simulink model "final_integration"  (R2019b)
settings: Solver=FixedStepDiscrete  StartTime=0.0  StopTime=100  FixedStep=0.1  RelTol=1e-3
undefined symbols (not defined in the file): DiscIntNeverNeededParam, gcbh, rmidispblock, sigbuilder_block
libraries: simulink x2
(part 1 of 2)
settings Model: Creator=User  LastModifiedBy=PRACHURJYA
settings OptimizationCC: DefaultParameterBehavior=Inlined  EnhancedBackFolding=on  PassReuseOutputArgsAs=Individual arguments  ZeroExternalMemoryAtStartup=off  ZeroInternalMemoryAtStartup=off  OptimizeBlockOrder=speed  DifferentSizesBufferReuse=on  OptimizationCustomize=off  EfficientTunableParamExpr=on
settings DebuggingCC: ParameterTunabilityLossMsg=error
settings SFSimCC: MATLABDynamicMemAlloc=off
settings RTWCC: SystemTargetFile=ert.tlc  TemplateMakefile=ert_default_tmf  GenerateReport=on  IncludeHyperlinkInReport=on  LaunchReport=on  GenerateTraceInfo=on  GenerateTraceReport=on  GenerateTraceReportSl=on  GenerateTraceReportSf=on  GenerateTraceReportEml=on
settings CodeAppCC: ForceParamTrailComments=on  IgnoreCustomStorageClasses=off  OperatorAnnotations=on  SimulinkDataObjDesc=on  SFDataObjDesc=on  InsertBlockDesc=on
settings ERTTargetCC: TargetLangStandard=C99 (ISO)  GenerateSampleERTMain=on  SupportContinuousTime=on  InlinedParameterPlacement=NonHierarchical  ERTCustomFileTemplate=example_file_process.tlc
settings ConfigComp: CovScope=ReferencedModels  CovMetricSettings=dcmwe  DVTestSuiteOptimization=Auto  DVDetectOutOfBounds=on

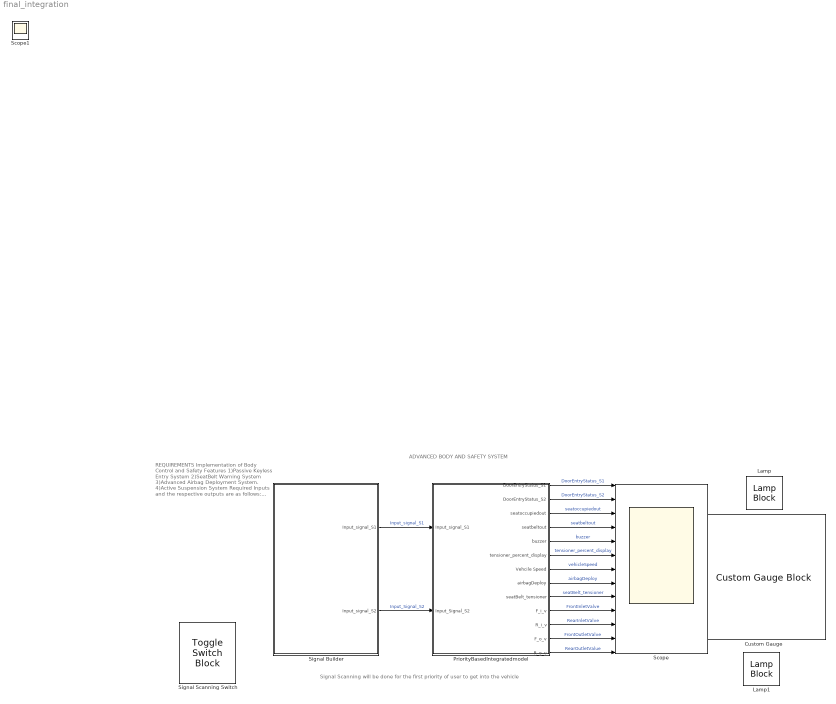
== system final_integration ==
  note: Signal Scanning will be done for the first priority of user to get into the vehicle
  note: REQUIREMENTS
      |
      | Implementation of Body Control and Safety Features
      | 1)Passive Keyless Entry System
      | 2)SeatBelt Warning System
      | 3)Advanced Airbag Deployment System.
      | 4)Active Suspension System
      |
      | Required Inputs and the respective outputs are as follows:
      | 1)Inputs: Input signal_s1
      | Input signal_s2
      | Ignition Status (on/off)
      | Seatbelt status (on/off)
      | Weight Sensor (kg)
      | Distance(cm)
      | Vehicle acceleration(m/s^2).
      | Pressure Input(psi)
      | Mode Status(0/1)
      |
      | 2)Outputs: DoorEntryStatus_S1
      | DoorEntryStatus_S2
      | Seat Occupied Status
      | SeatBelt Status
      | Tensioner Percent
      | Vehicle Speed
      | Airbag Deployment/Steering retraction
      | Seatbelt tensioner status
      | Front/Rear valve signals
  note: ADVANCED BODY AND SAFETY SYSTEM
  Custom Gauge : CustomGaugeBlock  LabelPosition=Bottom  NeedleImage=data:image/svg+xml;base64,PD94bWwgdmVyc2lvbj0iMS4wIiBlbmNvZGluZz0idXRmLTgiPz4KPCEtLSBHZW5lcmF0b3I6IEFkb2JlIElsbHVzdHJhdG9yIDE5LjIuMSwgU1ZHIEV4cG9ydCBQbHVnLUluIC4gU1ZHIFZlcnNpb246IDYuMDAgQnVpbGQgMCkgIC0tPgo8c3ZnIHZlcnNpb249IjEuMSIgeG1sbnM9Imh0dHA6Ly93d3cudzMub3JnLzIwMDAvc3ZnIiB4bWxuczp4bGluaz0iaHR0cDovL3d3dy53My5vcmcvMTk5OS94bGluayIgeD0iMHB4IiB5PSIwcHgiCgkgdmlld0JveD0iMCAwIDIwMCA1MCIgc3R5bGU9ImVuYWJsZS1iYWNrZ3JvdW5kOm5ldyAw ...(+9940 chars)  NeedleXPos=0.3848836610088748  NeedleYPos=0.4819046056238141  NeedleHeight=0.1115133381335879  NeedleWidth=0.18370999021718049  NeedleInitialRotation=-59.94322499147643  BackgroundImage=data:image/svg+xml;base64,PD94bWwgdmVyc2lvbj0iMS4wIiBlbmNvZGluZz0iVVRGLTgiIHN0YW5kYWxvbmU9Im5vIj8+CjwhLS0gR2VuZXJhdG9yOiBBZG9iZSBJbGx1c3RyYXRvciAxOS4yLjEsIFNWRyBFeHBvcnQgUGx1Zy1JbiAuIFNWRyBWZXJzaW9uOiA2LjAwIEJ1aWxkIDApICAtLT4KCjxzdmcKICAgeG1sbnM6ZGM9Imh0dHA6Ly9wdXJsLm9yZy9kYy9lbGVtZW50cy8xLjEvIgogICB4bWxuczpjYz0iaHR0cDovL2NyZWF0aXZlY29tbW9ucy5vcmcvbnMjIgogICB4bWxuczpyZGY9Imh0dHA6Ly93d3cudzMub3JnLzE5OTkvMDIvMjItcmRmLXN5bnRh ...(+9660 chars)  GaugeMax=35  GaugeArcDefined=true  GaugeArcRadius=0.13057749678689773  GaugeArcStrokeWidth=0.03818590063686888  GaugeArcRotation=240.5385250290321  GaugeArcRatio=0.8333333333333  GaugeArcTransparency=0  ValueArcColor=#1759b0  GaugeTickColor=#faf5c8  ScaleColorsJSON=[]  fixedAspectRatio=on  IsLinearGauge=false  GaugeTrackLeft=0.35  GaugeTrackTop=0.35  GaugeTrackHeight=0.1  GaugeTrackWidth=0.3  GaugeTrackRotation=0
  Lamp : LampBlock  LabelPosition=Bottom
  Lamp1 : LampBlock  LabelPosition=Bottom
  PriorityBasedIntegratedmodel : Subsystem
  Scope : Scope  NumInputPorts=13
  Signal Builder : Subsystem  Tag=STV Subsys  LoadFcn=sigbuilder_block('load');  StartFcn=sigbuilder_block('start');  StopFcn=sigbuilder_block('stop');  ClipboardFcn=sigbuilder_block('clipboard');  mask(Sigbuilder block){tuvar=[0:10]}
      mask help: Simulink:masks:SigbuilderBlock_MD
      mask init:
      | if ~strcmp(get_param(bdroot(gcbh),'SimulationStatus'),'stopped') tuvar = sigbuilder_block('maskInit'); end
      settings: CopyFcn=sigbuilder_block('copy');  DeleteFcn=sigbuilder_block('delete');  ModelCloseFcn=sigbuilder_block('modelClose');  PreSaveFcn=sigbuilder_block('preSave');  PauseFcn=sigbuilder_block('pause');  ContinueFcn=sigbuilder_block('continue');  NameChangeFcn=sigbuilder_block('namechange');  OpenFcn=sigbuilder_block('open',[0 30 1152 561.6 ]);  CloseFcn=sigbuilder_block('close');
      mask Display: plot(0, 0, 100, 100,[2, 2, 32, 32, 2], [68, 8, 8, 68, 68],[32, 2], [38, 38], [32, 19, 2],[53, 60, 44], [32, 17, 17, 2],[16, 16, 31, 31]);txt = getActiveGroup(gcbh);text(2, 100, txt,'verticalAlignment', 'top');
  Signal Scanning Switch : ToggleSwitchBlock  LabelPosition=Bottom
      settings: Values={{'Off', 'On'}, [0 1]}
  Scope1 : Scope
  wires:
  Signal Builder/1(Input_signal_S1) -> PriorityBasedIntegratedmodel/1(Input_signal_S1)  "Input_signal_S1"
  Signal Builder/2(Input_signal_S2) -> PriorityBasedIntegratedmodel/2(Input_Signal_S2)  "Input_Signal_S2"
  PriorityBasedIntegratedmodel/1(DoorEntryStatus_S1) -> Scope/1  "DoorEntryStatus_S1"
  PriorityBasedIntegratedmodel/2(DoorEntryStatus_S2) -> Scope/2  "DoorEntryStatus_S2"
  PriorityBasedIntegratedmodel/3(seatoccupiedout) -> Scope/3  "seatoccupiedout"
  PriorityBasedIntegratedmodel/4(seatbeltout) -> Scope/4  "seatbeltout"
  PriorityBasedIntegratedmodel/5(buzzer) -> Scope/5  "buzzer"
  PriorityBasedIntegratedmodel/6(tensioner_percent_display) -> Scope/6  "tensioner_percent_display"
  PriorityBasedIntegratedmodel/7(Vehcile Speed) -> Scope/7  "vehicleSpeed"
  PriorityBasedIntegratedmodel/8(airbagDeploy) -> Scope/8  "airbagDeploy"
  PriorityBasedIntegratedmodel/9(seatBelt_tensioner) -> Scope/9  "seatBelt_tensioner"
  PriorityBasedIntegratedmodel/10(F_i_v) -> Scope/10  "FrontInletValve"
  PriorityBasedIntegratedmodel/11(R_i_v) -> Scope/11  "RearInletValve"
  PriorityBasedIntegratedmodel/12(F_o_v) -> Scope/12  "FrontOutletValve"
  PriorityBasedIntegratedmodel/13(R_o_v) -> Scope/13  "RearOutletValue"

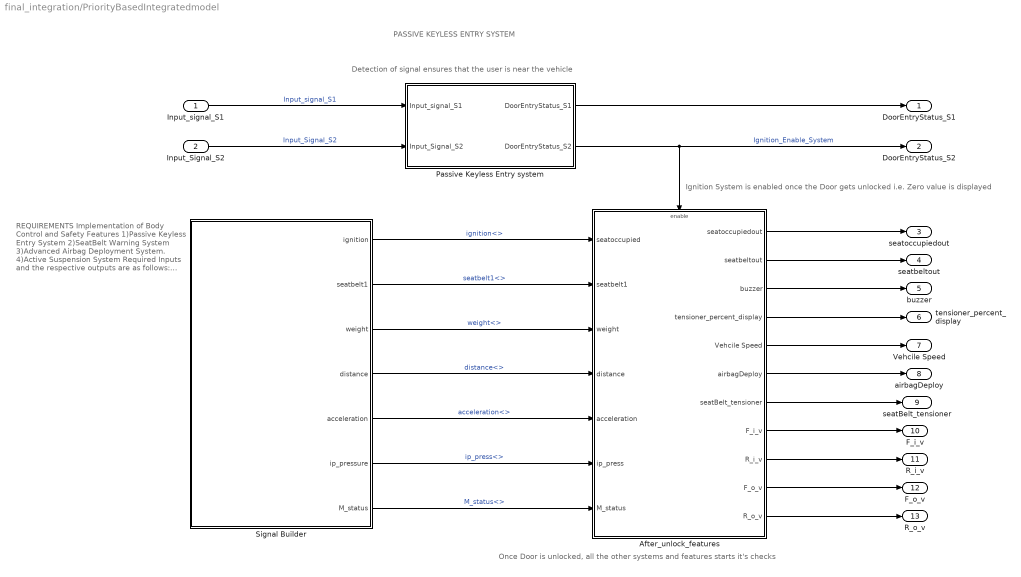
== system final_integration/PriorityBasedIntegratedmodel ==
  note: Once Door is unlocked, all the other systems and features starts it's checks
  note: Ignition System is enabled once the Door gets unlocked i.e. Zero value is displayed
  note: Detection of signal ensures that the user is near the vehicle
  note: PASSIVE KEYLESS ENTRY SYSTEM
  note: REQUIREMENTS
      |
      | Implementation of Body Control and Safety Features
      | 1)Passive Keyless Entry System
      | 2)SeatBelt Warning System
      | 3)Advanced Airbag Deployment System.
      | 4)Active Suspension System
      |
      | Required Inputs and the respective outputs are as follows:
      | 1)Inputs: Input signal_s1
      | Input signal_s2
      | Ignition Status (on/off)
      | Seatbelt status (on/off)
      | Weight Sensor (kg)
      | Distance(cm)
      | Vehicle acceleration(m/s^2).
      | Pressure Input(psi)
      | Mode Status(0/1)
      |
      | 2)Outputs: DoorEntryStatus_S1
      | DoorEntryStatus_S2
      | Seat Occupied Status
      | SeatBelt Status
      | Tensioner Percent
      | Vehicle Speed
      | Airbag Deployment/Steering retraction
      | Seatbelt tensioner status
      | Front/Rear valve signals
  Input_signal_S1 : Inport
  Input_Signal_S2 : Inport  Port=2
  "After_unlock_features " : Subsystem  TreatAsAtomicUnit=on
  Passive Keyless Entry system : Subsystem
  Signal Builder : Subsystem  Tag=STV Subsys  LoadFcn=sigbuilder_block('load');  StartFcn=sigbuilder_block('start');  StopFcn=sigbuilder_block('stop');  ClipboardFcn=sigbuilder_block('clipboard');  mask(Sigbuilder block){tuvar=[0:10]}
      mask help: Simulink:masks:SigbuilderBlock_MD
      mask init:
      | if ~strcmp(get_param(bdroot(gcbh),'SimulationStatus'),'stopped') tuvar = sigbuilder_block('maskInit'); end
      settings: CopyFcn=sigbuilder_block('copy');  DeleteFcn=sigbuilder_block('delete');  ModelCloseFcn=sigbuilder_block('modelClose');  PreSaveFcn=sigbuilder_block('preSave');  PauseFcn=sigbuilder_block('pause');  ContinueFcn=sigbuilder_block('continue');  NameChangeFcn=sigbuilder_block('namechange');  OpenFcn=sigbuilder_block('open',[0 30 1152 561.6 ]);  CloseFcn=sigbuilder_block('close');
      mask Display: plot(0, 0, 100, 100,[2, 2, 32, 32, 2], [68, 8, 8, 68, 68],[32, 2], [38, 38], [32, 19, 2],[53, 60, 44], [32, 17, 17, 2],[16, 16, 31, 31]);txt = getActiveGroup(gcbh);text(2, 100, txt,'verticalAlignment', 'top');
  DoorEntryStatus_S1 : Outport
  DoorEntryStatus_S2 : Outport  Port=2
  seatoccupiedout : Outport  Port=3
  seatbeltout : Outport  Port=4
  buzzer : Outport  Port=5
  tensioner_percent_display : Outport  Port=6
  Vehcile Speed : Outport  Port=7
  airbagDeploy : Outport  Port=8
  seatBelt_tensioner : Outport  Port=9
  F_i_v : Outport  Port=10
  R_i_v : Outport  Port=11
  F_o_v : Outport  Port=12
  R_o_v : Outport  Port=13
  wires:
  "After_unlock_features "/1(seatoccupiedout) -> seatoccupiedout/1
  "After_unlock_features "/2(seatbeltout) -> seatbeltout/1
  "After_unlock_features "/3(buzzer) -> buzzer/1
  "After_unlock_features "/4(tensioner_percent_display) -> tensioner_percent_display/1
  "After_unlock_features "/5(Vehcile Speed) -> Vehcile Speed/1
  "After_unlock_features "/6(airbagDeploy) -> airbagDeploy/1
  "After_unlock_features "/7(seatBelt_tensioner) -> seatBelt_tensioner/1
  "After_unlock_features "/8(F_i_v) -> F_i_v/1
  "After_unlock_features "/9(R_i_v) -> R_i_v/1
  "After_unlock_features "/10(F_o_v) -> F_o_v/1
  "After_unlock_features "/11(R_o_v) -> R_o_v/1
  Passive Keyless Entry system/1(DoorEntryStatus_S1) -> DoorEntryStatus_S1/1
  Input_signal_S1/1 -> Passive Keyless Entry system/1(Input_signal_S1)  "Input_signal_S1"
  Input_Signal_S2/1 -> Passive Keyless Entry system/2(Input_Signal_S2)  "Input_Signal_S2"
  Passive Keyless Entry system/2(DoorEntryStatus_S2) -> "After_unlock_features "/Enable, DoorEntryStatus_S2/1  "Ignition_Enable_System"
  Signal Builder/1(ignition) -> "After_unlock_features "/1(seatoccupied)  "ignition<>"
  Signal Builder/7(M_status) -> "After_unlock_features "/7(M_status)  "M_status<>"
  Signal Builder/2(seatbelt1) -> "After_unlock_features "/2(seatbelt1)  "seatbelt1<>"
  Signal Builder/4(distance) -> "After_unlock_features "/4(distance)  "distance<>"
  Signal Builder/5(acceleration) -> "After_unlock_features "/5(acceleration)  "acceleration<>"
  Signal Builder/6(ip_pressure) -> "After_unlock_features "/6(ip_press)  "ip_press<>"
  Signal Builder/3(weight) -> "After_unlock_features "/3(weight)  "weight<>"

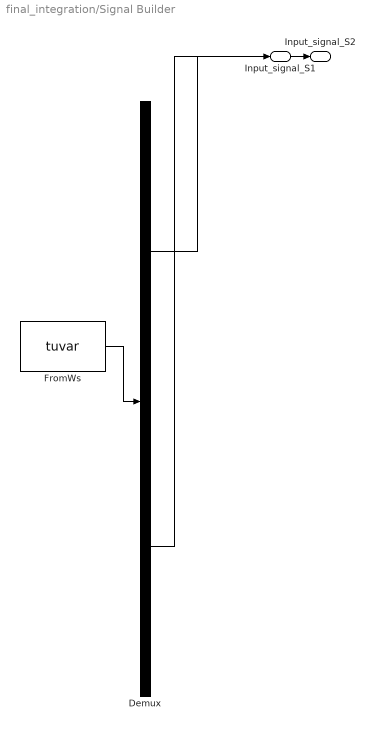
== system final_integration/Signal Builder ==
  Demux : Demux  Tag=STV Demux  Outputs=2
  FromWs : FromWorkspace  Tag=STV FromWs  VariableName=tuvar  SampleTime=0
      SigBuilderData=|
      | common.afterFinalStr = 'Extrapolate'
      | common.sampleTime = 0
      | dataSet.timeRange = [0 100]
      | dataSet.name = 'Passive_entry_system_Signals'
      | sbobj.Groups.Name = 'Passive_entry_system_Signals'
      | sbobj.Groups.Signals(1).Name = 'Input_signal_S1'
      | sbobj.Groups.Signals(1).XData = [0 0.96 7.5 10 100]
      | sbobj.Groups.Signals(1).YData = [0 100 750 1000 1000]
      | sbobj.Groups.Signals(2).Name = 'Input_signal_S2'
      | sbobj.Groups.Signals(2).XData = [0 4 6.16 10 100]
      | sbobj.Groups.Signals(2).YData = [1000 600 384 0 0]
      | sbobj.Groups.TimeRange = [0 100]
  Input_signal_S1 : Outport  Tag=STV Outport
  Input_signal_S2 : Outport  Tag=STV Outport  Port=2
  wires:
  FromWs/1 -> Demux/1
  Demux/1 -> Input_signal_S1/1
  Demux/2 -> Input_signal_S2/1

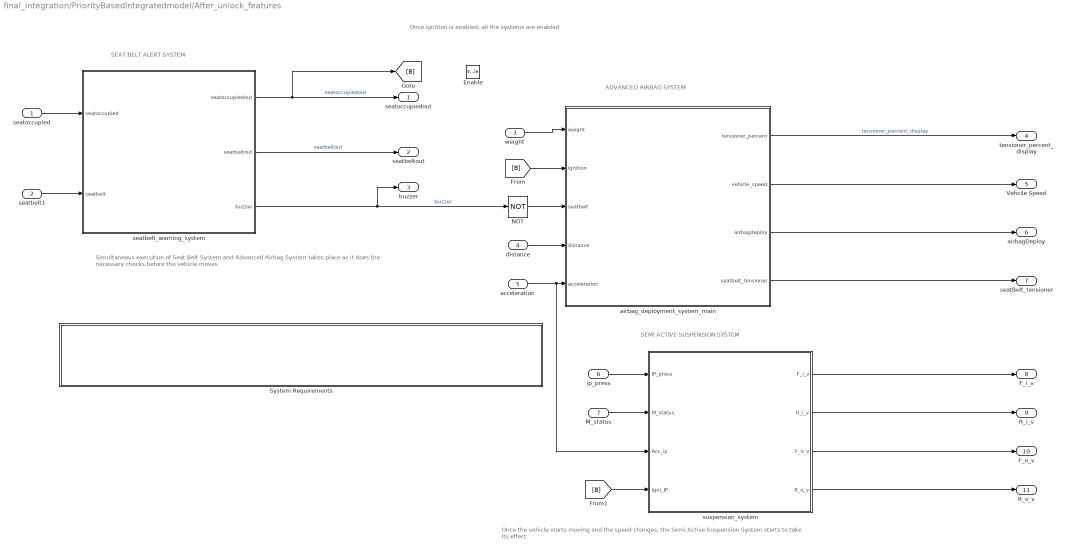
== system final_integration/PriorityBasedIntegratedmodel/After_unlock_features  ==
  note: Once the vehicle starts moving and the speed changes, the Semi Active Suspension System starts to take its effect
  note: Simultaneous execution of Seat Belt System and Advanced Airbag System takes place as
      | it does the necessary checks before the vehicle moves
  note: Once ignition is enabled, all the systems are enabled
  note: SEAT BELT ALERT SYSTEM
  note: ADVANCED AIRBAG SYSTEM
  note: SEMI ACTIVE SUSPENSION SYSTEM
  seatoccupied : Inport
  seatbelt1 : Inport  Port=2
  weight : Inport  Port=3
  distance : Inport  Port=4
  acceleration : Inport  Port=5
  ip_press : Inport  Port=6
  M_status : Inport  Port=7
  Enable : EnablePort
  NOT : Logic  Operator=NOT  IconShape=distinctive  AllPortsSameDT=off  OutDataTypeStr=boolean
  System Requirements : Subsystem  LoadFcn=rmidispblock('load',gcbh)  mask(System Requirements){id=SystemReq, title=System Requirements}
      mask prompts: title "Block Title"
      mask help: Lists the requirements for the current model.
      mask init:
      | id = 'SystemReq';
      | [w,h] = rmidispblock('display',gcbh);
      settings: CopyFcn=rmidispblock('create',gcbh)  DeleteFcn=rmidispblock('delete',gcbh)  ModelCloseFcn=rmidispblock('close',gcbh)  PreSaveFcn=rmidispblock('close',gcbh)  PostSaveFcn=rmidispblock('open',gcbh)  OpenFcn=rmidispblock('open',gcbh)  MoveFcn=rmidispblock('move',gcbh)
      mask Help: helpview(fullfile(docroot,'slrequirements','helptargets.map'),'systemrequirements')
      mask Display: text(746/2,93-4,rmidispblock('title',gcbh),'horizontalAlignment','center','verticalAlignment','top')
  airbag_deployment_system_main : Subsystem
  seatbelt_warning_system : Subsystem
  suspension_system : Subsystem
  seatoccupiedout : Outport
  seatbeltout : Outport  Port=2
  buzzer : Outport  Port=3
  tensioner_percent_display : Outport  Port=4
  Vehcile Speed : Outport  Port=5
  airbagDeploy : Outport  Port=6
  seatBelt_tensioner : Outport  Port=7
  F_i_v : Outport  Port=8
  R_i_v : Outport  Port=9
  F_o_v : Outport  Port=10
  R_o_v : Outport  Port=11
  wires:
  seatbelt1/1 -> seatbelt_warning_system/2(seatbelt)
  seatbelt_warning_system/2(seatbeltout) -> seatbeltout/1  "seatbeltout"
  seatoccupied/1 -> seatbelt_warning_system/1(seatoccupied)
  seatbelt_warning_system/1(seatoccupiedout) -> [B], seatoccupiedout/1  "seatoccupiedout"
  seatbelt_warning_system/3(buzzer) -> buzzer/1, NOT/1  "buzzer"
  distance/1 -> airbag_deployment_system_main/4(distance)
  weight/1 -> airbag_deployment_system_main/1(weight)
  airbag_deployment_system_main/4(seatbelt_tensioner) -> seatBelt_tensioner/1
  NOT/1 -> airbag_deployment_system_main/3(seatbelt)
  airbag_deployment_system_main/3(airbagdeploy) -> airbagDeploy/1
  airbag_deployment_system_main/2(vehicle_speed) -> Vehcile Speed/1
  airbag_deployment_system_main/1(tensioner_percent) -> tensioner_percent_display/1  "tensioner_percent_display"
  [B] -> airbag_deployment_system_main/2(ignition)
  suspension_system/4(R_o_v) -> R_o_v/1
  [B] -> suspension_system/4(Igni_IP)
  suspension_system/2(R_i_v) -> R_i_v/1
  ip_press/1 -> suspension_system/1(IP_press)
  suspension_system/1(F_i_v) -> F_i_v/1
  suspension_system/3(F_o_v) -> F_o_v/1
  M_status/1 -> suspension_system/2(M_status)
  acceleration/1 -> suspension_system/3(Acc_ip), airbag_deployment_system_main/5(acceleration)

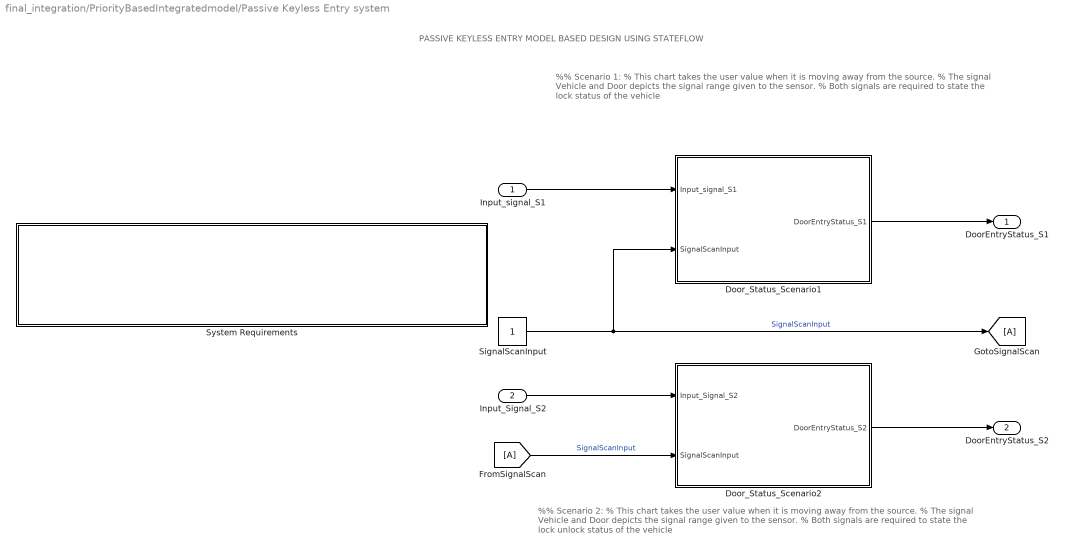
== system final_integration/PriorityBasedIntegratedmodel/Passive Keyless Entry system ==
  note: PASSIVE KEYLESS ENTRY MODEL BASED DESIGN USING STATEFLOW
  note: %% Scenario 1:
      | % This chart takes the user value when it is moving away from the source.
      | % The signal Vehicle and Door depicts the signal range given to the sensor.
      | % Both signals are required to state the lock status of the vehicle
  note: %% Scenario 2:
      | % This chart takes the user value when it is moving away from the source.
      | % The signal Vehicle and Door depicts the signal range given to the sensor.
      | % Both signals are required to state the lock unlock status of the vehicle
  Input_signal_S1 : Inport
  Input_Signal_S2 : Inport  Port=2
  Door_Status_Scenario1 : Stateflow chart  TreatAsAtomicUnit=on
  Door_Status_Scenario2 : Stateflow chart  TreatAsAtomicUnit=on
  SignalScanInput : Constant
  System Requirements : Subsystem  LoadFcn=rmidispblock('load',gcbh)  mask(System Requirements){id=SystemReq, title=System Requirements}
      mask prompts: title "Block Title"
      mask help: Lists the requirements for the current model.
      mask init:
      | id = 'SystemReq';
      | [w,h] = rmidispblock('display',gcbh);
      settings: CopyFcn=rmidispblock('create',gcbh)  DeleteFcn=rmidispblock('delete',gcbh)  ModelCloseFcn=rmidispblock('close',gcbh)  PreSaveFcn=rmidispblock('close',gcbh)  PostSaveFcn=rmidispblock('open',gcbh)  OpenFcn=rmidispblock('open',gcbh)  MoveFcn=rmidispblock('move',gcbh)
      mask Help: helpview(fullfile(docroot,'slrequirements','helptargets.map'),'systemrequirements')
      mask Display: text(511/2,108-4,rmidispblock('title',gcbh),'horizontalAlignment','center','verticalAlignment','top')
  DoorEntryStatus_S1 : Outport
  DoorEntryStatus_S2 : Outport  Port=2
  wires:
  Door_Status_Scenario1/1(DoorEntryStatus_S1) -> DoorEntryStatus_S1/1
  SignalScanInput/1 -> Door_Status_Scenario1/2(SignalScanInput), [A]  "SignalScanInput"
  Door_Status_Scenario2/1(DoorEntryStatus_S2) -> DoorEntryStatus_S2/1
  Input_signal_S1/1 -> Door_Status_Scenario1/1(Input_signal_S1)
  Input_Signal_S2/1 -> Door_Status_Scenario2/1(Input_Signal_S2)
  [A] -> Door_Status_Scenario2/2(SignalScanInput)  "SignalScanInput"

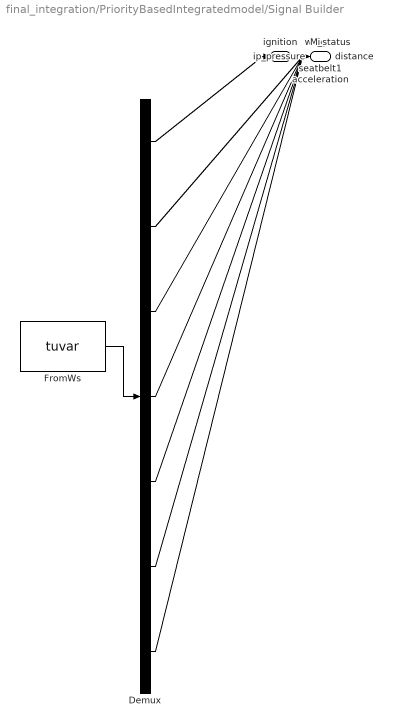
== system final_integration/PriorityBasedIntegratedmodel/Signal Builder ==
  Demux : Demux  Tag=STV Demux  Outputs=7
  FromWs : FromWorkspace  Tag=STV FromWs  VariableName=tuvar  SampleTime=0
      SigBuilderData=|
      | common.afterFinalStr = 'Extrapolate'
      | common.sampleTime = 0
      | dataSet.timeRange = [0 100]
      | dataSet.name = 'Passive_entry_system_Signals'
      | sbobj.Groups.Name = 'Passive_entry_system_Signals'
      | sbobj.Groups.Signals(1).Name = 'ignition'
      | sbobj.Groups.Signals(1).XData = [0 1 2 3 4 5 6 7 7 8 9 9 10 11 11 12 13 13 14 15 16 17 18 19 20 21 22 23 24 25 26 27 28 29 30 31 31.5 31.9 32.3 32.7 33.1 33.5 33.9 34.3 34.7 35.1 35.5 35.9 36.3 36.7 37.1 37.5 37.9 38.3 39 40 41 42 43 44 45 46 47 48 49 50 51 52 53 54 55 56 57 58 59 60 61 62 63 64 65 66 67 68 69 70 71 72 73 74 75 76 77 77 78 79 80 81 82 83 84 85 86 87 88 89 90 91 92 93 94 95 96 97 98 99 100]
      | sbobj.Groups.Signals(1).YData = [0 0 0 1 1 1 1 1 0 0 0 1 1 1 0 0 0 1 1 1 1 1 1 1 1 1 1 1 1 1 1 1 1 1 1 1 0 0 0 0 0 0 0 0 0 0 0 0 0 0 0 0 0 0 0 1 1 1 1 1 1 0 1 1 1 1 0 1 1 0 1 1 1 0 1 1 1 1 1 1 1 1 1 1 0 0 1 0 1 1 1 1 1 0 0 1 1 1 1 1 1 0 1 1 1 1 0 1 1 0 1 1 1 1 1 1 1]
      | sbobj.Groups.Signals(2).Name = 'seatbelt1'
      | sbobj.Groups.Signals(2).XData = [0 1 2 3 3 4 4 5 6 7 7 8 9 10 11 12 13 13 14 15 16 17 18 18 19 20 21 22 23 24 25 26 27 28 29 30 31 31 31.5 31.9 32.3 32.7 33.1 33.5 33.9 34.3 34.7 35.1 35.5 35.9 36.3 36.7 37.1 37.5 37.9 38.3 39 40 40 41 42 43 44 45 46 47 48 49 50 50 51 52 53 54 55 56 57 58 59 60 60 61 62 63 64 65 66 67 68 69 70 71 72 73 73 74 74 75 76 77 77 78 79 79 80 81 82 83 84 85 86 87 88 89 89 90 91 92 93 94 95 95 96 97 98 99 100]
      | sbobj.Groups.Signals(2).YData = [0 0 0 0 1 1 0 0 0 0 1 1 1 1 1 1 1 0 0 0 0 0 0 1 1 1 1 1 1 1 1 1 1 1 1 1 1 0 0 0 1 1 1 1 1 1 1 1 1 1 1 1 1 1 1 1 1 1 0 0 1 1 1 1 1 1 1 1 1 0 0 1 1 1 1 1 1 1 1 1 0 0 1 1 1 1 1 1 1 1 0 1 0 0 1 1 0 0 0 0 1 1 1 0 0 1 1 1 1 1 1 1 1 1 0 0 1 1 1 1 0 1 1 1 1 1 1]
      | sbobj.Groups.Signals(3).Name = 'weight'
      | sbobj.Groups.Signals(3).XData = [0 1 1 2 2 3 3 4 4 5 5 6 6 7 7 8 8 9 9 10 10 11 11 12 12 13 13 14 14 15 15 16 16 17 17 18 18 19 19 20 20 21 21 22 23 24 24 25 25 26 26 27 27 28 28 29 29 30 30 31 31 31.5 31.9 32.3 32.7 33.1 33.5 33.9 34.3 34.7 35.1 35.5 35.9 36.3 36.7 37.1 37.5 37.9 38.3 39 40 41 42 43 44 45 46 47 48 49 50 51 52 52 53 53 54 55 56 57 58 58 59 60 60 61 62 63 63 64 64 65 65 66 66 67 67 68 68 69 70 71 71 72 73 73 74 74 75 75 76 76 77 77 78 78 79 80 81 82 83 84 85 86 87 88 89 90 91 91 92 92 93 94 95 95 96 97 98 99 100]
      | sbobj.Groups.Signals(3).YData = [78 78 68 66 55 55 87 87 43 43 30 30 20 20 10 10 70 70 88 88 99 99 66 66 54 54 34 34 44 44 89 89 86 86 10 10 54 54 44 44 99 99 75 106 106 50 25 25 33 33 26 26 57 57 78 78 57 57 78 78 86 10 10 54 54 44 44 99 99 75 106 106 106 106 50 25 25 33 33 66 55 87 43 30 20 10 70 88 99 66 54 34 44 78 78 86 10 54 44 99 75 106 106 106 50 25 33 66 78 86 10 10 54 54 44 44 99 99 75 106 78 44 99 55 55 87 87 43 43 30 30 20 20 10 10 70 55 87 43 30 20 10 70 88 99 66 54 34 44 78 78 86 10 106 50 86 10 54 44 99 75]
      | sbobj.Groups.Signals(4).Name = 'distance'
      | sbobj.Groups.Signals(4).XData = [0 1 2 3 4 5 6 7 8 9 10 11 12 13 14 15 16 17 18 19 20 21 22 23 24 25 26 27 28 29 30 31 31 31.5 31.9 32.3 32.7 33.1 33.5 33.9 34.3 34.7 35.1 35.5 35.9 36.3 36.7 37.1 37.5 37.9 38.3 39 40 40 41 41 42 42 43 43 44 44 45 45 46 46 47 47 48 48 49 49 50 51 52 53 54 55 56 57 58 59 60 60 61 61 62 62 63 63 64 64 65 65 66 66 67 67 68 68 69 69 70 70 71 71 72 73 74 75 76 77 78 79 79 80 80 81 81 82 82 83 83 84 84 85 85 86 86 87 87 88 88 89 90 91 92 93 94 94 95 95 96 97 98 99 100]
      | sbobj.Groups.Signals(4).YData = [21 22 24 10 18 23 29 50 23 16 13 21 22 19 14 24 15 19 11 22 17 22 24 10 18 23 29 50 23 50 23 23 19 19 11 11 22 22 17 17 22 22 24 24 10 10 18 18 23 23 29 17 17 22 22 24 24 10 10 18 18 23 23 29 29 50 50 23 23 50 50 23 23 19 11 22 17 22 24 10 18 23 29 17 17 22 22 24 24 10 10 18 18 23 23 29 29 50 50 23 23 50 21 22 29 50 24 10 18 23 29 50 23 17 22 22 24 24 10 10 18 18 23 23 29 29 50 50 23 23 50 50 23 23 19 11 22 17 23 29 17 10 18 23 29 50 23]
      | sbobj.Groups.Signals(5).Name = 'acceleration'
      | sbobj.Groups.Signals(5).XData = [0 1 2 3 4 5 6 7 8 9 10 11 12 13 14 15 16 17 18 19 20 21 22 23 24 25 26 27 28 29 30 31 31 31.5 31.9 32.3 32.7 33.1 33.5 33.9 34.3 34.7 35.1 35.5 35.9 36.3 36.7 37.1 37.5 37.9 38.3 39 40 41 42 43 44 45 46 47 48 49 50 51 52 53 54 55 56 57 58 59 60 61 62 63 64 65 66 67 68 69 69 70 70 71 72 73 74 75 76 77 78 79 80 81 82 83 84 85 86 87 88 89 90 91 92 93 94 94 95 95 96 96 97 97 98 98 99 99 100]
      | sbobj.Groups.Signals(5).YData = [9 12 45 54 67 12 47 34 67 23 89 23 52 9 76 13 67 34 90 28 49 12 45 54 67 12 47 34 67 34 67 67 34 34 90 90 90 90 90 90 90 90 90 45 54 54 67 67 12 12 47 12 45 54 67 20 50 34 67 23 89 23 52 76 50 13 67 45 14 88 49 42 45 24 67 12 99 34 67 50 99 9 12 9 12 50 45 54 67 12 47 34 67 45 54 67 20 50 34 67 23 89 23 52 76 50 13 67 42 45 45 99 99 34 34 67 67 50 50 99 99]
      | sbobj.Groups.Signals(6).Name = 'ip_pressure'
      | sbobj.Groups.Signals(6).XData = [0 1 2 3 4 5 6 7 8 9 10 11 12 13 14 15 16 17 18 19 20 21 22 23 24 25 26 27 28 29 30 31 31 31.5 31.9 32.3 32.7 33.1 33.5 33.9 34.3 34.7 35.1 35.5 35.9 36.3 36.7 37.1 37.5 37.9 38.3 39 40 41 42 43 44 45 46 47 48 49 50 51 52 53 54 55 56 57 58 59 60 61 62 63 64 65 66 67 68 69 69 70 70 71 72 73 74 75 76 77 78 79 80 81 82 83 84 85 86 87 88 89 90 91 92 93 94 94 95 96 97 97 98 99 99 100]
      | sbobj.Groups.Signals(6).YData = [-100 -80 60 45 65 100 76 23 98 45 119 102 99 66 34 56 22 97 67 9 78 -80 60 45 65 100 76 23 98 23 0 0 97 97 67 67 9 9 78 78 -80 -80 60 60 45 45 65 65 100 100 76 -50 -10 10 30 50 50 100 110 100 40 80 140 50 50 15 17 100 100 100 88 100 50 50 44 66 50 50 100 100 50 -100 -50 -100 -80 100 60 45 65 100 76 23 98 -10 10 30 50 50 100 110 100 40 80 140 50 50 15 17 100 50 50 50 50 100 100 100 50 50]
      | sbobj.Groups.Signals(7).Name = 'M_status'
      | sbobj.Groups.Signals(7).XData = [0 1 2 2 3 4 5 6 7 7 8 9 9 10 11 11 12 13 13 14 15 16 17 18 19 20 21 22 22 23 24 25 26 27 27 28 29 30 31 31.5 31.9 32.3 32.7 33.1 33.5 33.9 34.3 34.7 35.1 35.5 35.9 36.3 36.7 37.1 37.5 37.9 38.3 39 40 41 42 43 44 45 46 47 48 49 50 51 52 53 54 55 56 57 58 59 60 61 62 63 64 65 66 67 68 69 70 71 72 73 74 75 76 77 77 78 79 80 81 82 83 84 85 86 87 88 89 90 91 92 93 94 94 95 96 97 97 98 99 99 100]
      | sbobj.Groups.Signals(7).YData = [0 0 0 1 1 1 1 1 1 0 0 0 1 1 1 0 0 0 1 1 1 1 1 1 1 1 0 0 1 1 1 1 1 1 0 0 1 1 1 1 1 1 1 1 1 1 0 0 0 1 1 1 1 1 1 1 1 0 1 1 1 0 0 1 1 1 0 0 0 0 0 0 0 1 1 1 0 1 0 0 0 0 0 0 1 1 0 0 0 1 1 1 1 1 1 1 0 0 1 1 1 0 0 1 1 1 0 0 0 0 0 0 0 1 0 0 0 0 1 1 1 0 0]
      | sbobj.Groups.TimeRange = [0 100]
  ignition : Outport  Tag=STV Outport
  seatbelt1 : Outport  Tag=STV Outport  Port=2
  weight : Outport  Tag=STV Outport  Port=3
  distance : Outport  Tag=STV Outport  Port=4
  acceleration : Outport  Tag=STV Outport  Port=5
  ip_pressure : Outport  Tag=STV Outport  Port=6
  M_status : Outport  Tag=STV Outport  Port=7
  wires:
  FromWs/1 -> Demux/1
  Demux/1 -> ignition/1
  Demux/2 -> seatbelt1/1
  Demux/3 -> weight/1
  Demux/4 -> distance/1
  Demux/5 -> acceleration/1
  Demux/6 -> ip_pressure/1
  Demux/7 -> M_status/1

== system final_integration/PriorityBasedIntegratedmodel/After_unlock_features /System Requirements ==
  Subsystem : Subsystem  mask{label=0, index=1}
      mask init:
      | label = rmidispblock('label',index);
      settings: OpenFcn=rmidispblock('openReq',gcbh);
      mask Display: text(0,0,label,'horizontalAlignment','left','verticalAlignment','bottom')

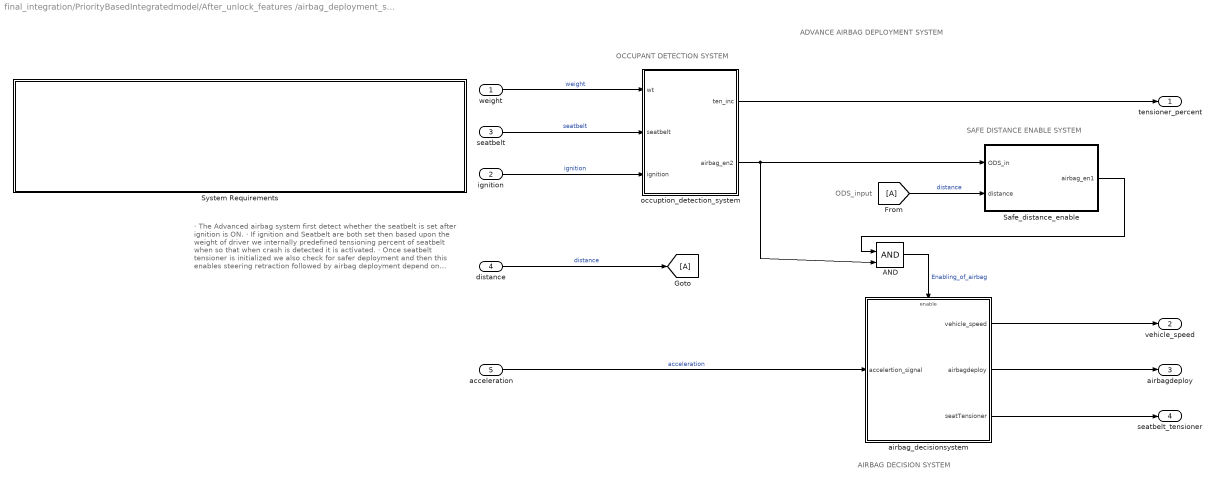
== system final_integration/PriorityBasedIntegratedmodel/After_unlock_features /airbag_deployment_system_main ==
  note: · The Advanced airbag system first detect whether the seatbelt is set after ignition is ON.
      | · If ignition and Seatbelt are both set then based upon the weight of driver we internally predefined tensioning percent of seatbelt when so that when crash is detected it is activated.
      | · Once seatbelt tensioner is initialized we also check for safer deployment and then this enables steering retraction followed by airbag deployment depend on crash level decided using vehicle acceleration
  note: ADVANCE AIRBAG DEPLOYMENT SYSTEM
  note: ODS_input
  note: OCCUPANT DETECTION SYSTEM
  note: SAFE DISTANCE ENABLE SYSTEM
  note: AIRBAG DECISION SYSTEM
  weight : Inport
  ignition : Inport  Port=2
  seatbelt : Inport  Port=3
  distance : Inport  Port=4
  acceleration : Inport  Port=5
  AND : Logic  IconShape=distinctive  AllPortsSameDT=off  OutDataTypeStr=boolean
  Safe_distance_enable : Subsystem
  System Requirements : Subsystem  LoadFcn=rmidispblock('load',gcbh)  mask(System Requirements){id=SystemReq, title=System Requirements}
      mask prompts: title "Block Title"
      mask help: Lists the requirements for the current model.
      mask init:
      | id = 'SystemReq';
      | [w,h] = rmidispblock('display',gcbh);
      settings: CopyFcn=rmidispblock('create',gcbh)  DeleteFcn=rmidispblock('delete',gcbh)  ModelCloseFcn=rmidispblock('close',gcbh)  PreSaveFcn=rmidispblock('close',gcbh)  PostSaveFcn=rmidispblock('open',gcbh)  OpenFcn=rmidispblock('open',gcbh)  MoveFcn=rmidispblock('move',gcbh)
      mask Help: helpview(fullfile(docroot,'slrequirements','helptargets.map'),'systemrequirements')
      mask Display: text(586/2,143-4,rmidispblock('title',gcbh),'horizontalAlignment','center','verticalAlignment','top')
  airbag_decisionsystem : Subsystem
  occuption_detection_system : Subsystem
  tensioner_percent : Outport
  vehicle_speed : Outport  Port=2
  airbagdeploy : Outport  Port=3
  seatbelt_tensioner : Outport  Port=4
  wires:
  occuption_detection_system/2(airbag_en2) -> Safe_distance_enable/1(ODS_in), AND/2
  distance/1 -> [A]  "distance"
  acceleration/1 -> airbag_decisionsystem/1(accelertion_signal)  "acceleration"
  airbag_decisionsystem/2(airbagdeploy) -> airbagdeploy/1
  [A] -> Safe_distance_enable/2(distance)  "distance"
  airbag_decisionsystem/3(seatTensioner) -> seatbelt_tensioner/1
  airbag_decisionsystem/1(vehicle_speed) -> vehicle_speed/1
  occuption_detection_system/1(ten_inc) -> tensioner_percent/1
  weight/1 -> occuption_detection_system/1(wt)  "weight"
  ignition/1 -> occuption_detection_system/3(ignition)  "ignition"
  seatbelt/1 -> occuption_detection_system/2(seatbelt)  "seatbelt"
  Safe_distance_enable/1(airbag_en1) -> AND/1
  AND/1 -> airbag_decisionsystem/Enable  "Enabling_of_airbag"

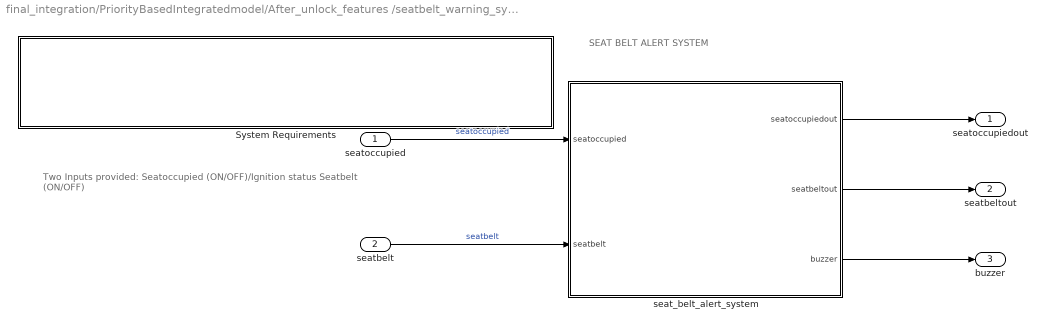
== system final_integration/PriorityBasedIntegratedmodel/After_unlock_features /seatbelt_warning_system ==
  note: Two Inputs provided:
      | Seatoccupied (ON/OFF)/Ignition status
      | Seatbelt (ON/OFF)
  note: SEAT BELT ALERT SYSTEM
  seatoccupied : Inport
  seatbelt : Inport  Port=2
  System Requirements : Subsystem  LoadFcn=rmidispblock('load',gcbh)  mask(System Requirements){id=SystemReq, title=System Requirements}
      mask prompts: title "Block Title"
      mask help: Lists the requirements for the current model.
      mask init:
      | id = 'SystemReq';
      | [w,h] = rmidispblock('display',gcbh);
      settings: CopyFcn=rmidispblock('create',gcbh)  DeleteFcn=rmidispblock('delete',gcbh)  ModelCloseFcn=rmidispblock('close',gcbh)  PreSaveFcn=rmidispblock('close',gcbh)  PostSaveFcn=rmidispblock('open',gcbh)  OpenFcn=rmidispblock('open',gcbh)  MoveFcn=rmidispblock('move',gcbh)
      mask Help: helpview(fullfile(docroot,'slrequirements','helptargets.map'),'systemrequirements')
      mask Display: text(531/2,88-4,rmidispblock('title',gcbh),'horizontalAlignment','center','verticalAlignment','top')
  seat_belt_alert_system : Stateflow chart  TreatAsAtomicUnit=on
  seatoccupiedout : Outport
  seatbeltout : Outport  Port=2
  buzzer : Outport  Port=3
  wires:
  seatoccupied/1 -> seat_belt_alert_system/1(seatoccupied)  "seatoccupied"
  seat_belt_alert_system/2(seatbeltout) -> seatbeltout/1
  seatbelt/1 -> seat_belt_alert_system/2(seatbelt)  "seatbelt"
  seat_belt_alert_system/3(buzzer) -> buzzer/1
  seat_belt_alert_system/1(seatoccupiedout) -> seatoccupiedout/1

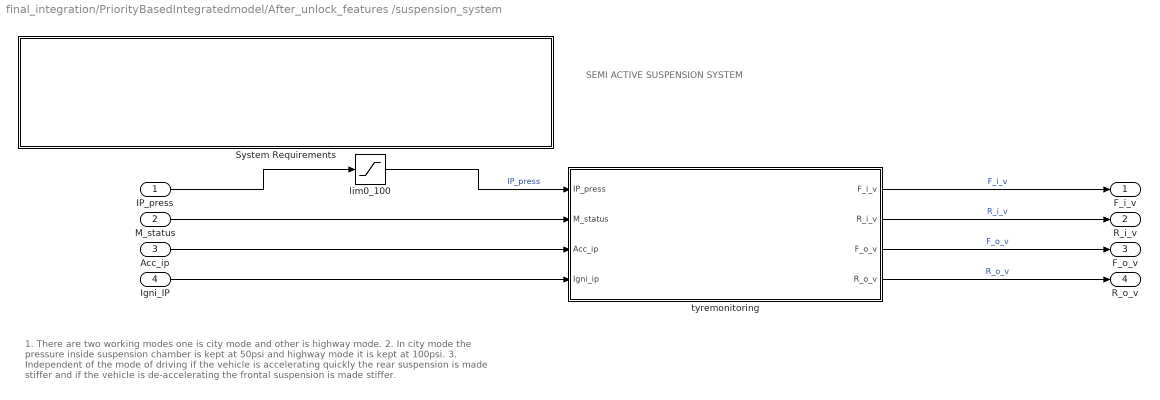
== system final_integration/PriorityBasedIntegratedmodel/After_unlock_features /suspension_system ==
  note: 1. There are two working modes one is city mode and other is highway mode.
      | 2. In city mode the pressure inside suspension chamber is kept at 50psi and highway mode it is kept at 100psi.
      | 3. Independent of the mode of driving if the vehicle is accelerating quickly the rear suspension is made stiffer and if the vehicle is de-accelerating the frontal suspension is made stiffer.
  note: SEMI ACTIVE SUSPENSION SYSTEM
  IP_press : Inport
  M_status : Inport  Port=2
  Acc_ip : Inport  Port=3
  Igni_IP : Inport  Port=4
  System Requirements : Subsystem  LoadFcn=rmidispblock('load',gcbh)  mask(System Requirements){id=SystemReq, title=System Requirements}
      mask prompts: title "Block Title"
      mask help: Lists the requirements for the current model.
      mask init:
      | id = 'SystemReq';
      | [w,h] = rmidispblock('display',gcbh);
      settings: CopyFcn=rmidispblock('create',gcbh)  DeleteFcn=rmidispblock('delete',gcbh)  ModelCloseFcn=rmidispblock('close',gcbh)  PreSaveFcn=rmidispblock('close',gcbh)  PostSaveFcn=rmidispblock('open',gcbh)  OpenFcn=rmidispblock('open',gcbh)  MoveFcn=rmidispblock('move',gcbh)
      mask Help: helpview(fullfile(docroot,'slrequirements','helptargets.map'),'systemrequirements')
      mask Display: text(531/2,108-4,rmidispblock('title',gcbh),'horizontalAlignment','center','verticalAlignment','top')
  lim0_100 : Saturate  UpperLimit=120  LowerLimit=0
      settings: AttributesFormatString=|
      | %<LowerLimit>=0
      | %<UpperLimit>=120
  tyremonitoring : Stateflow chart  TreatAsAtomicUnit=on
  F_i_v : Outport
  R_i_v : Outport  Port=2
  F_o_v : Outport  Port=3
  R_o_v : Outport  Port=4
  wires:
  tyremonitoring/2(R_i_v) -> R_i_v/1  "R_i_v"
  tyremonitoring/4(R_o_v) -> R_o_v/1  "R_o_v"
  tyremonitoring/1(F_i_v) -> F_i_v/1  "F_i_v"
  lim0_100/1 -> tyremonitoring/1(IP_press)  "IP_press"
  Acc_ip/1 -> tyremonitoring/3(Acc_ip)
  M_status/1 -> tyremonitoring/2(M_status)
  tyremonitoring/3(F_o_v) -> F_o_v/1  "F_o_v"
  Igni_IP/1 -> tyremonitoring/4(Igni_ip)
  IP_press/1 -> lim0_100/1

== system final_integration/PriorityBasedIntegratedmodel/Passive Keyless Entry system/System Requirements ==
  Subsystem : Subsystem  mask{label=0, index=1}
      mask init:
      | label = rmidispblock('label',index);
      settings: OpenFcn=rmidispblock('openReq',gcbh);
      mask Display: text(0,0,label,'horizontalAlignment','left','verticalAlignment','bottom')

== system final_integration/PriorityBasedIntegratedmodel/After_unlock_features /System Requirements/Subsystem ==

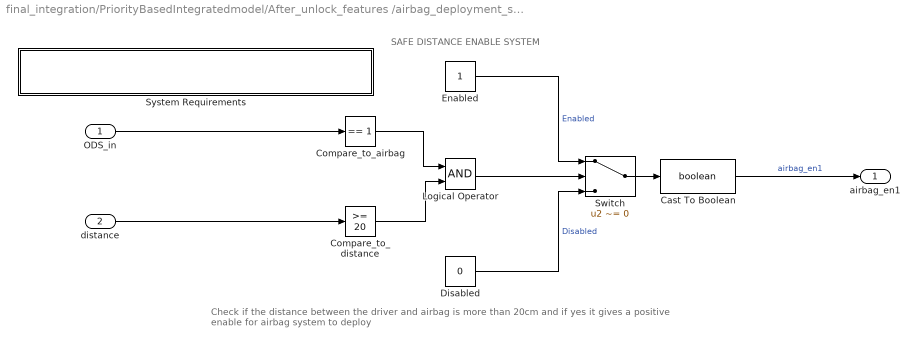
== system final_integration/PriorityBasedIntegratedmodel/After_unlock_features /airbag_deployment_system_main/Safe_distance_enable ==
  note: Check if the distance between the driver and airbag is more than 20cm and if yes it gives a positive enable for airbag system to deploy
  note: SAFE DISTANCE ENABLE SYSTEM
  ODS_in : Inport
  distance : Inport  Port=2
  Cast To Boolean : DataTypeConversion  OutDataTypeStr=boolean
  Compare_to_airbag : simulink/Logic and Bit Operations/Compare To Constant  relop===  const=1  OutDataTypeStr=boolean
  Compare_to_distance : simulink/Logic and Bit Operations/Compare To Constant  relop=>=  const=20  OutDataTypeStr=boolean
  Disabled : Constant  Value=0
  Enabled : Constant
  Logical Operator : Logic  AllPortsSameDT=off  OutDataTypeStr=boolean
  Switch : Switch  Criteria=u2 ~= 0
  System Requirements : Subsystem  LoadFcn=rmidispblock('load',gcbh)  mask(System Requirements){id=SystemReq, title=System Requirements}
      mask prompts: title "Block Title"
      mask help: Lists the requirements for the current model.
      mask init:
      | id = 'SystemReq';
      | [w,h] = rmidispblock('display',gcbh);
      settings: CopyFcn=rmidispblock('create',gcbh)  DeleteFcn=rmidispblock('delete',gcbh)  ModelCloseFcn=rmidispblock('close',gcbh)  PreSaveFcn=rmidispblock('close',gcbh)  PostSaveFcn=rmidispblock('open',gcbh)  OpenFcn=rmidispblock('open',gcbh)  MoveFcn=rmidispblock('move',gcbh)
      mask Help: helpview(fullfile(docroot,'slrequirements','helptargets.map'),'systemrequirements')
      mask Display: text(351/2,43-4,rmidispblock('title',gcbh),'horizontalAlignment','center','verticalAlignment','top')
  airbag_en1 : Outport  OutDataTypeStr=boolean
  wires:
  distance/1 -> Compare_to_distance/1
  Compare_to_distance/1 -> Logical Operator/2
  ODS_in/1 -> Compare_to_airbag/1
  Logical Operator/1 -> Switch/2
  Disabled/1 -> Switch/3  "Disabled"
  Enabled/1 -> Switch/1  "Enabled"
  Compare_to_airbag/1 -> Logical Operator/1
  Switch/1 -> Cast To Boolean/1
  Cast To Boolean/1 -> airbag_en1/1  "airbag_en1"

== system final_integration/PriorityBasedIntegratedmodel/After_unlock_features /airbag_deployment_system_main/System Requirements ==
  Subsystem : Subsystem  mask{label=0, index=1}
      mask init:
      | label = rmidispblock('label',index);
      settings: OpenFcn=rmidispblock('openReq',gcbh);
      mask Display: text(0,0,label,'horizontalAlignment','left','verticalAlignment','bottom')

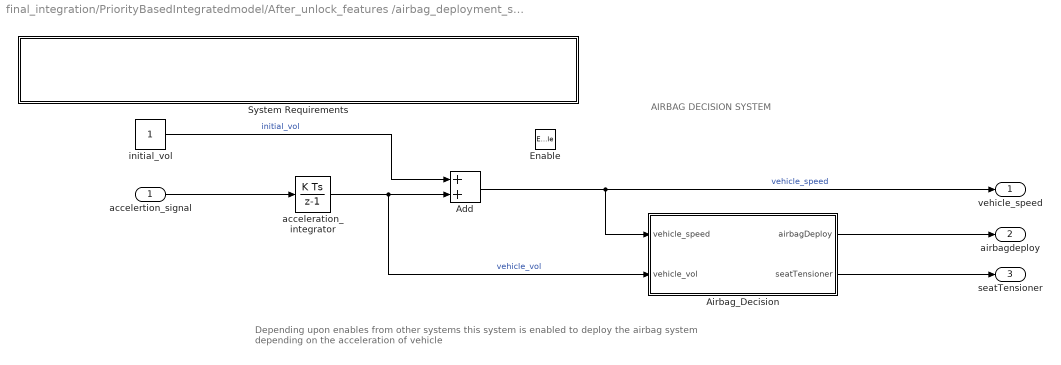
== system final_integration/PriorityBasedIntegratedmodel/After_unlock_features /airbag_deployment_system_main/airbag_decisionsystem ==
  note: Depending upon enables from other systems this system is enabled to deploy the airbag system depending on the acceleration of vehicle
  note: AIRBAG DECISION SYSTEM
  accelertion_signal : Inport
  Enable : EnablePort
  Add : Sum
  Airbag_Decision : Stateflow chart  TreatAsAtomicUnit=on
  System Requirements : Subsystem  LoadFcn=rmidispblock('load',gcbh)  mask(System Requirements){id=SystemReq, title=System Requirements}
      mask prompts: title "Block Title"
      mask help: Lists the requirements for the current model.
      mask init:
      | id = 'SystemReq';
      | [w,h] = rmidispblock('display',gcbh);
      settings: CopyFcn=rmidispblock('create',gcbh)  DeleteFcn=rmidispblock('delete',gcbh)  ModelCloseFcn=rmidispblock('close',gcbh)  PreSaveFcn=rmidispblock('close',gcbh)  PostSaveFcn=rmidispblock('open',gcbh)  OpenFcn=rmidispblock('open',gcbh)  MoveFcn=rmidispblock('move',gcbh)
      mask Help: helpview(fullfile(docroot,'slrequirements','helptargets.map'),'systemrequirements')
      mask Display: text(556/2,63-4,rmidispblock('title',gcbh),'horizontalAlignment','center','verticalAlignment','top')
  acceleration_integrator : DiscreteIntegrator  SampleTime=-1  ICPrevOutput=DiscIntNeverNeededParam  ICPrevScaledInput=DiscIntNeverNeededParam
  initial_vol : Constant
  vehicle_speed : Outport
  airbagdeploy : Outport  Port=2
  seatTensioner : Outport  Port=3
  wires:
  Add/1 -> vehicle_speed/1, Airbag_Decision/1(vehicle_speed)  "vehicle_speed"
  Airbag_Decision/1(airbagDeploy) -> airbagdeploy/1
  Airbag_Decision/2(seatTensioner) -> seatTensioner/1
  initial_vol/1 -> Add/1  "initial_vol"
  accelertion_signal/1 -> acceleration_integrator/1
  acceleration_integrator/1 -> Add/2, Airbag_Decision/2(vehicle_vol)  "vehicle_vol"
